simulink model "attitude_comp_filter"  (R2023a)
settings: configuration reference "configuration_filter" (kept outside this file)
undefined symbols (not defined in the file): correction_performed_bool, DiscIntNeverNeededParam, Eul_rad, filt, rot_K_est_OB_B_radDs, sfor_est_B_mDs, sim
libraries: lib_kinematics x1, lib_others x1
settings Model: Creator=FC_dev1  LastModifiedBy=FC_dev1
settings ConfigSetRef: SourceName=configuration_filter  SourceLocation=Base Workspace

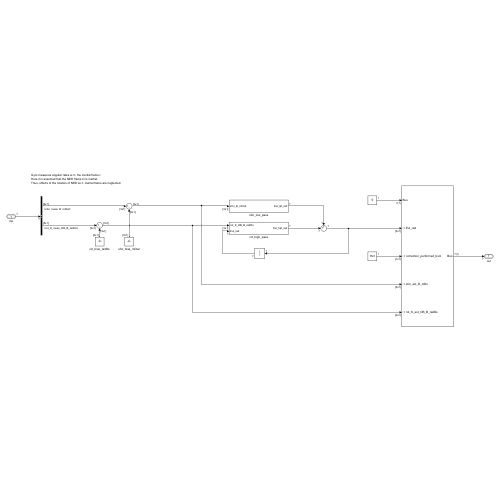
[thumbnail: Simulink's stored preview of the top-level diagram]
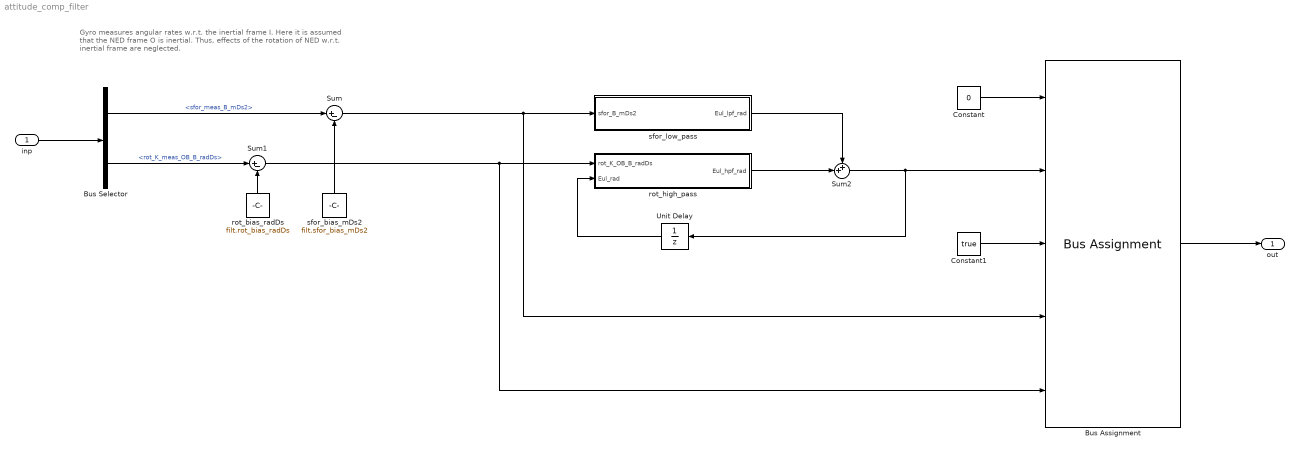
== system attitude_comp_filter ==
  note: Gyro measures angular rates w.r.t. the inertial frame I.
      | Here it is assumed that the NED frame O is inertial.
      | Thus, effects of the rotation of NED w.r.t. inertial frame are neglected.
  inp : Inport  OutDataTypeStr=Bus: inp_Bus
  Bus Assignment : BusAssignment  AssignedSignals=Eul_rad,correction_performed_bool,sfor_est_B_mDs,rot_K_est_OB_B_radDs
  Bus Selector : BusSelector  OutputSignals=sfor_meas_B_mDs2,rot_K_meas_OB_B_radDs
  Constant : Constant  Value=0  OutDataTypeStr=Bus: out_Bus
  Constant1 : Constant  Value=true
  Sum : Sum  Inputs=|+-
  Sum1 : Sum  Inputs=|+-
  Sum2 : Sum  Inputs=++|
  Unit Delay : UnitDelay  SampleTime=-1  HasFrameUpgradeWarning=on
  rot_bias_radDs : Constant  Value=filt.rot_bias_radDs  VectorParams1D=off
  rot_high_pass : Subsystem
  sfor_bias_mDs2 : Constant  Value=filt.sfor_bias_mDs2  VectorParams1D=off
  sfor_low_pass : Subsystem
  out : Outport  OutDataTypeStr=Bus: out_Bus
  wires:
  Bus Selector/1 -> Sum/1  "<sfor_meas_B_mDs2>"
  Bus Selector/2 -> Sum1/1  "<rot_K_meas_OB_B_radDs>"
  Constant/1 -> Bus Assignment/1
  Bus Assignment/1 -> out/1
  inp/1 -> Bus Selector/1
  rot_bias_radDs/1 -> Sum1/2
  sfor_bias_mDs2/1 -> Sum/2
  Sum/1 -> Bus Assignment/4, sfor_low_pass/1(sfor_B_mDs2)
  Sum1/1 -> Bus Assignment/5, rot_high_pass/1(rot_K_OB_B_radDs)
  rot_high_pass/1(Eul_hpf_rad) -> Sum2/2
  Sum2/1 -> Bus Assignment/2, Unit Delay/1
  sfor_low_pass/1(Eul_lpf_rad) -> Sum2/1
  Constant1/1 -> Bus Assignment/3
  Unit Delay/1 -> rot_high_pass/2(Eul_rad)

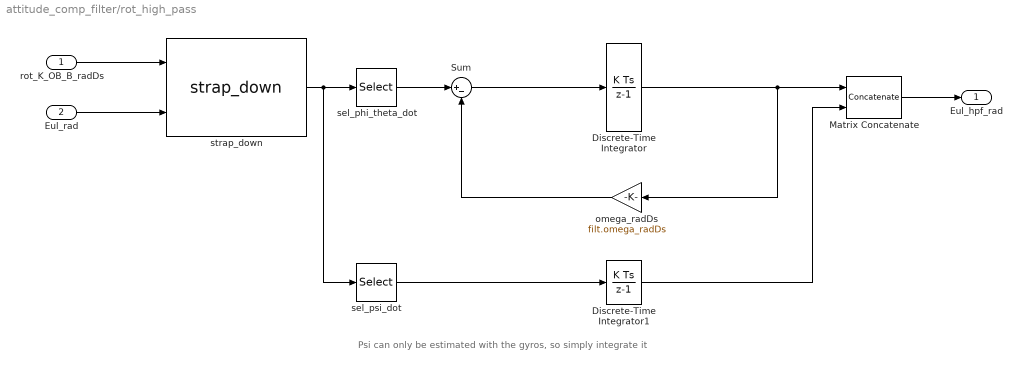
== system attitude_comp_filter/rot_high_pass ==
  note: Psi can only be estimated with the gyros, so simply integrate it
  rot_K_OB_B_radDs : Inport
  Eul_rad : Inport  Port=2
  Discrete-Time Integrator : DiscreteIntegrator  SampleTime=sim.sample_time_s  ICPrevOutput=DiscIntNeverNeededParam  ICPrevScaledInput=DiscIntNeverNeededParam
  Discrete-Time Integrator1 : DiscreteIntegrator  SampleTime=sim.sample_time_s  ICPrevOutput=DiscIntNeverNeededParam  ICPrevScaledInput=DiscIntNeverNeededParam
  Matrix Concatenate : Concatenate  Mode=Multidimensional array
  Sum : Sum  Inputs=|+-
  omega_radDs : Gain  Gain=filt.omega_radDs
  sel_phi_theta_dot : Selector  NumberOfDimensions=2  InputPortWidth=3  IndexOptions=Index vector (dialog),Index vector (dialog)  Indices=[1 2],1  OutputSizes=1,1
  sel_psi_dot : Selector  NumberOfDimensions=2  InputPortWidth=3  IndexOptions=Index vector (dialog),Index vector (dialog)  Indices=3,1  OutputSizes=1,1
  strap_down : lib_kinematics/strap_down  SystemSampleTime=-1  VariantActivationTime=update diagram  Latency=0  AutoFrameSizeCalculation=off
  Eul_hpf_rad : Outport
  wires:
  Discrete-Time Integrator/1 -> omega_radDs/1, Matrix Concatenate/1
  Sum/1 -> Discrete-Time Integrator/1
  rot_K_OB_B_radDs/1 -> strap_down/1
  Eul_rad/1 -> strap_down/2
  omega_radDs/1 -> Sum/2
  strap_down/1 -> sel_psi_dot/1, sel_phi_theta_dot/1
  sel_phi_theta_dot/1 -> Sum/1
  sel_psi_dot/1 -> Discrete-Time Integrator1/1
  Matrix Concatenate/1 -> Eul_hpf_rad/1
  Discrete-Time Integrator1/1 -> Matrix Concatenate/2

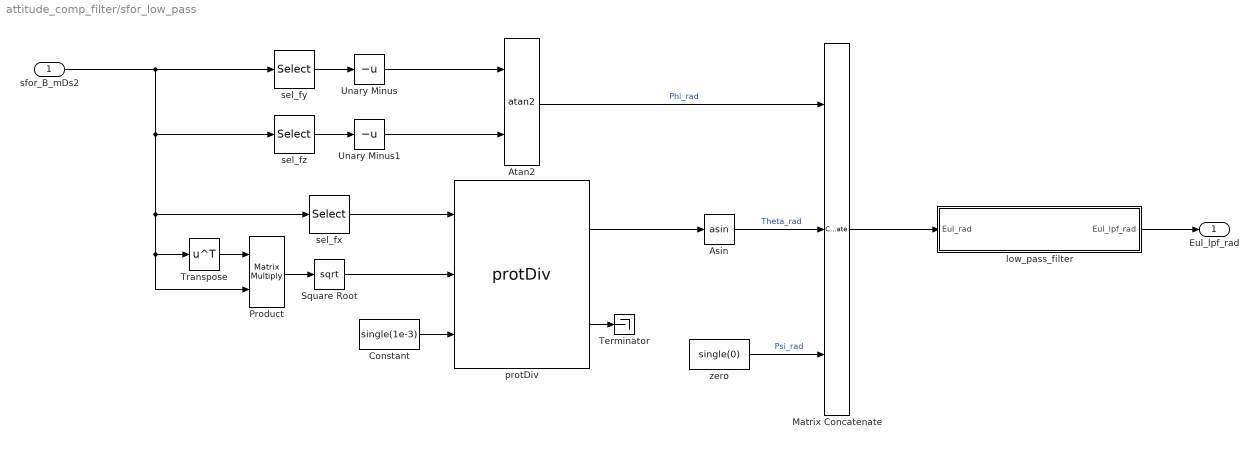
== system attitude_comp_filter/sfor_low_pass ==
  sfor_B_mDs2 : Inport
  Asin : Trigonometry  Operator=asin
  Atan2 : Trigonometry  Operator=atan2
  Constant : Constant  Value=single(1e-3)
  Matrix Concatenate : Concatenate  NumInputs=3  Mode=Multidimensional array
  Product : Product  Multiplication=Matrix(*)
  Square Root : Sqrt
  Terminator : Terminator
  Transpose : Math  Operator=transpose
  Unary Minus : UnaryMinus
  Unary Minus1 : UnaryMinus
  low_pass_filter : Subsystem
  protDiv : lib_others/protDiv  SystemSampleTime=-1  VariantActivationTime=update diagram  Latency=0  AutoFrameSizeCalculation=off
  sel_fx : Selector  NumberOfDimensions=2  InputPortWidth=3  IndexOptions=Index vector (dialog),Index vector (dialog)  Indices=1,1  OutputSizes=1,1
  sel_fy : Selector  NumberOfDimensions=2  InputPortWidth=3  IndexOptions=Index vector (dialog),Index vector (dialog)  Indices=2,1  OutputSizes=1,1
  sel_fz : Selector  NumberOfDimensions=2  InputPortWidth=3  IndexOptions=Index vector (dialog),Index vector (dialog)  Indices=3,1  OutputSizes=1,1
  zero : Constant  Value=single(0)
  Eul_lpf_rad : Outport
  wires:
  sfor_B_mDs2/1 -> sel_fz/1, Product/2, Transpose/1, sel_fx/1, sel_fy/1
  Transpose/1 -> Product/1
  Product/1 -> Square Root/1
  Square Root/1 -> protDiv/2
  sel_fx/1 -> protDiv/1
  protDiv/1 -> Asin/1
  protDiv/2 -> Terminator/1
  Constant/1 -> protDiv/3
  Unary Minus/1 -> Atan2/1
  sel_fy/1 -> Unary Minus/1
  sel_fz/1 -> Unary Minus1/1
  Unary Minus1/1 -> Atan2/2
  Asin/1 -> Matrix Concatenate/2  "Theta_rad"
  Atan2/1 -> Matrix Concatenate/1  "Phi_rad"
  zero/1 -> Matrix Concatenate/3  "Psi_rad"
  low_pass_filter/1(Eul_lpf_rad) -> Eul_lpf_rad/1
  Matrix Concatenate/1 -> low_pass_filter/1(Eul_rad)

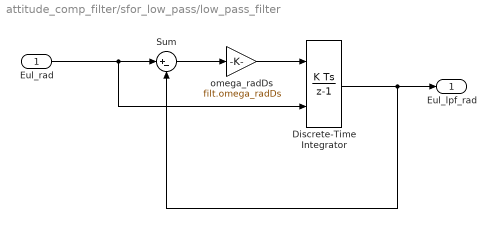
== system attitude_comp_filter/sfor_low_pass/low_pass_filter ==
  Eul_rad : Inport
  Discrete-Time Integrator : DiscreteIntegrator  InitialConditionSource=external  SampleTime=sim.sample_time_s  ICPrevOutput=DiscIntNeverNeededParam  ICPrevScaledInput=DiscIntNeverNeededParam
  Sum : Sum  Inputs=|+-
  omega_radDs : Gain  Gain=filt.omega_radDs
  Eul_lpf_rad : Outport
  wires:
  omega_radDs/1 -> Discrete-Time Integrator/1
  Discrete-Time Integrator/1 -> Eul_lpf_rad/1, Sum/2
  Sum/1 -> omega_radDs/1
  Eul_rad/1 -> Sum/1, Discrete-Time Integrator/2
